simulink model "Hover_ITAE_prefilter"  (Simulink 6.6)
settings: Solver=ode45  StartTime=0.0  StopTime=10.0  RelTol=1e-3
settings Model: Creator=user  LastModifiedBy=user

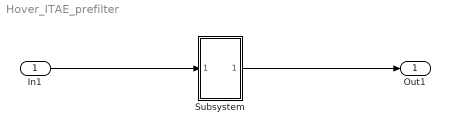
== system Hover_ITAE_prefilter ==
  In1 : Inport
  Subsystem : Subsystem
  Out1 : Outport
  wires:
  In1/1 -> Subsystem/1(In1)
  Subsystem/1(Out1) -> Out1/1

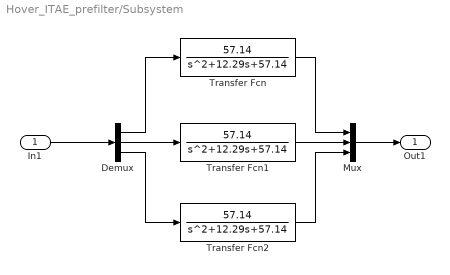
== system Hover_ITAE_prefilter/Subsystem ==
  In1 : Inport
  Demux : Demux  Outputs=3
  Mux : Mux  Inputs=3
  Transfer Fcn : TransferFcn  Numerator=[57.14]  Denominator="[1  12.29 57.14]"
  Transfer Fcn1 : TransferFcn  Numerator=[57.14]  Denominator="[1  12.29 57.14]"
  Transfer Fcn2 : TransferFcn  Numerator=[57.14]  Denominator="[1  12.29 57.14]"
  Out1 : Outport
  wires:
  Mux/1 -> Out1/1
  Transfer Fcn1/1 -> Mux/2
  Transfer Fcn/1 -> Mux/1
  Transfer Fcn2/1 -> Mux/3
  Demux/1 -> Transfer Fcn/1
  Demux/2 -> Transfer Fcn1/1
  Demux/3 -> Transfer Fcn2/1
  In1/1 -> Demux/1
